simulink model "sine_table"  (Simulink 7.9)
settings: Solver=FixedStepDiscrete  SolverMode=SingleTasking  StartTime=0.0  StopTime=10.0  RelTol=1e-3
libraries: shlslibv1 x5
settings Model: synDspstartup=OK  Creator=sszilvasi  LastModifiedBy=sszilvasi
settings DataIOCC: SaveOutput=off  SignalLogging=off  SaveTime=off
settings OptimizationCC: InlineParams=on
settings DebuggingCC: AlgebraicLoopMsg=error

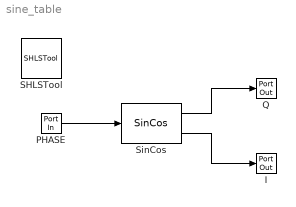
== system sine_table ==
  I : shlslibv1/Ports & Subsystems/Port Out  syn_capture=off  syn_register=on  synBlockType=port  synLatency=1  synBlockId=1
  PHASE : shlslibv1/Ports & Subsystems/Port In  syn_out_wl=12  syn_out_fl=11  syn_out_dt=signed  syn_out_st=1  syn_capture=off  syn_register=on  syn_out_sat=off  syn_out_rnd=off  synBlockType=port  synLatency=1  synBlockId=0
  Q : shlslibv1/Ports & Subsystems/Port Out  syn_capture=off  syn_register=on  synBlockType=port  synLatency=1  synBlockId=1
  SHLSTool : shlslibv1/SHLSTool  synBlockType=tool  syn_dsp_mode=FPGA
  SinCos : shlslibv1/Math Functions/SinCos  syn_sincos_opr=sin&cos  syn_sincos_amp=.999  syn_out_f=Specify  syn_out_wl=10  syn_out_fl=8  synBlockType=primitive  synLatency=1  synBlockId=65
  wires:
  PHASE/1 -> SinCos/1
  SinCos/1 -> Q/1
  SinCos/2 -> I/1
